simulink model "AC_DC"  (R2022b)
settings: Solver=FixedStepDiscrete  StartTime=0.0  StopTime=2  FixedStep=1e-6  RelTol=1e-3
libraries: spsRMSLib x11, spsSeriesRLCBranchLib x9, simulink x7, spsVoltageMeasurementLib x7, spsCurrentMeasurementLib x6, spsMosfetLib x6, spsIdealSwitchLib x3, spsFourierLib x2, spsMeanLib x2, slpidlib x2, sps_lib x1, spsControlledVoltageSourceLib x1
(part 1 of 2)
settings Model: SimulationMode=accelerator  Creator=XIAO  LastModifiedBy=XIAO
settings SolverCC: AutoInsertRateTranBlk=on
settings DataIOCC: ReturnWorkspaceOutputs=off

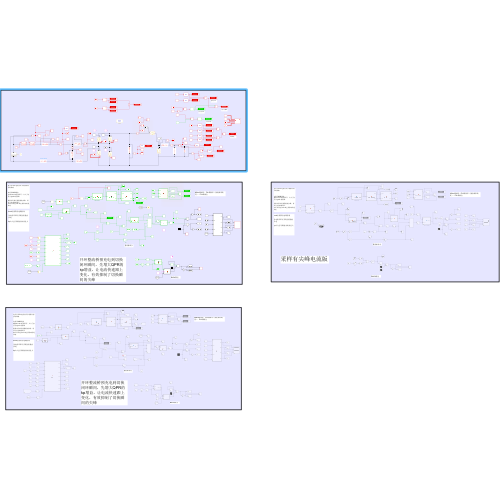
[thumbnail: Simulink's stored preview of the top-level diagram]
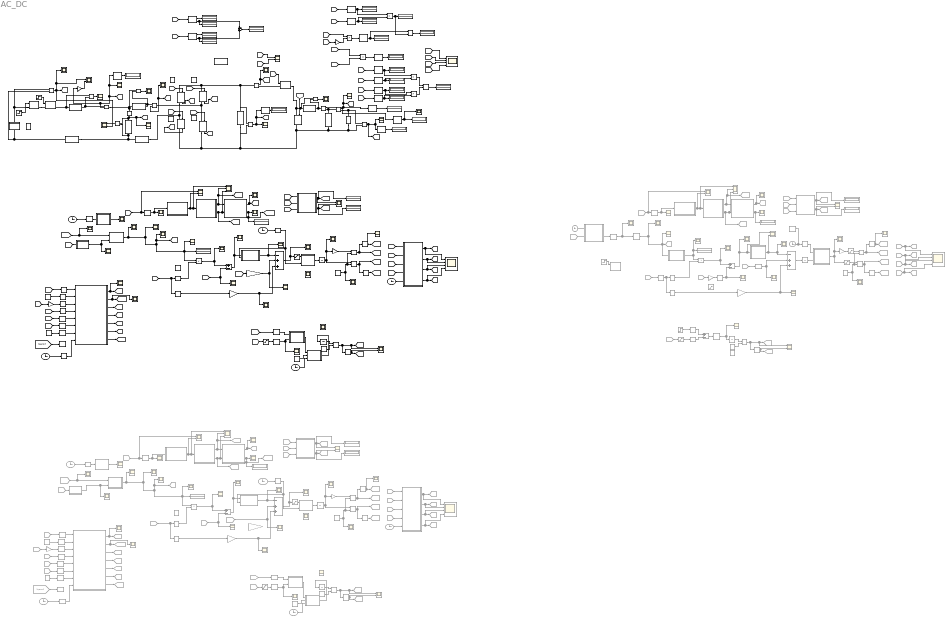
== system AC_DC ==
  note: BUCK降压
  note: buck恒流降压电路控制
      |
      | 单电流环即可实现恒流输出供电
      |
      | kp太大会导致输出纹波过大
  note: 功率因数PF
  note: 有功功率P
  note: 无功功率Q
  note: 视在功率s
  note: 电压外环PI 电流内环多谐振比例控制策略
      |
      | 电流环QPR调参
      | kp在0.2~0.3范围即可，太大了容易引起LCL谐振峰
      |
      | 根据实际情况调整谐波参数，谐波大对应kr就调大
      | wc可以固定在6~10主要影响的是带宽
  note: 效率η
  note: 整流桥部分
  note: 20khz锁相环，FLL锁频率（预防频率畸变），PLL锁相位
  note: 采样有尖峰电流版本
  note: 电压外环PI 电流内环多谐振比例控制策略
      |
      | 电流环QPR调参
      | kp在0.2~0.3范围即可，太大了容易引起LCL谐振峰
      |
      | 根据实际情况调整谐波参数，谐波大对应kr就调大
      | wc可以固定在6~10主要影响的是带宽
  note: buck恒流降压电路控制
      |
      | 单电流环即可实现恒流输出供电
      |
      | kp太大会导致输出纹波过大
  note: BUCK降压
  note: 整流桥部分
  note: 20khz锁相环，FLL锁频率（预防频率畸变），PLL锁相位
  note: 开环整流桥预充电到切换闭环瞬间，先增大QPR的kp增益，让电流快速跟上变化，有效抑制了切换瞬间的尖峰
  note: 电压外环PI 电流内环多谐振比例控制策略
      |
      | 电流环QPR调参
      | kp在0.2~0.3范围即可，太大了容易引起LCL谐振峰
      |
      | 根据实际情况调整谐波参数，谐波大对应kr就调大
      | wc可以固定在6~10主要影响的是带宽
  note: buck恒流降压电路控制
      |
      | 单电流环即可实现恒流输出供电
      |
      | kp太大会导致输出纹波过大
  note: BUCK降压
  note: 20khz锁相环，FLL锁频率（预防频率畸变），PLL锁相位
  note: 整流桥部分
  note: 开环整流桥预充电到切换闭环瞬间，先增大QPR的kp增益，让电流快速跟上变化，有效抑制了切换瞬间的尖峰
  -ug4 : Saturate  Commented=on  UpperLimit=1  LowerLimit=-1
  Add1 : Sum  Commented=on  Inputs=+-
  Add10 : Sum  Commented=on  Inputs=+-
  Add12 : Sum  Commented=on  Inputs=-++
  Add2 : Sum  Commented=on  Inputs=+-
  Add3 : Sum  Commented=on  Inputs=-++
  Add4 : Sum  Inputs=+-
  Add9 : Sum  Inputs=-++
  Clock{1..5} (5 alike) : Clock
  Clock{6..12} (7 alike) : Clock  Commented=on
  Constant{,4..6,8} (5 alike) : Constant  Value=0
  Constant1 : Constant  Commented=on  Value=0
  Constant10 : Constant  Commented=on  Value=55
  Constant11 : Constant  Commented=on
  Constant2 : Constant  Value=4.365
  Constant3 : Constant  Value=55
  Constant7 : Constant  Value=2
  Constant9 : Constant  Commented=on  Value=4.365
  Cos1 : Trigonometry  Operator=cos
  Cos2 : Trigonometry
  Cos3 : Trigonometry  Commented=on  Operator=cos
  Cos4 : Trigonometry  Commented=on
  Cos6 : Trigonometry  Commented=on  Operator=cos
  Cos7 : Trigonometry  Commented=on
  Current Measurement{1..6} (6 alike) : spsCurrentMeasurementLib/Current Measurement  PhasorSimulation=off  OutputType=Complex  PSBequivalent=0
  Display{,1..4,6..18,22,26..31} (25 alike) : Display
  Display{5,19..21,23,32..34} (8 alike) : Display  Commented=on
  Divide : Product  Inputs=*/
  Divide1 : Product  Inputs=/*
  Fourier7 : spsFourierLib/Fourier  Freq=50  n=1  InInit=[0, 0]  Ts=1e-6
  Fourier8 : spsFourierLib/Fourier  Freq=50  n=1  InInit=[0, 0]  Ts=1e-6
  From{19,41..42,55} (4 alike) : From  Commented=on  GotoTag=theta
  From43 : From  Commented=on  GotoTag=ua
  From{44,58,64,71} (4 alike) : From  Commented=on  GotoTag=Uref
  From45 : From  Commented=on  GotoTag=u_alpha
  From46 : From  Commented=on  GotoTag=u_beta
  From47 : From  Commented=on  GotoTag=IL2_
  From48 : From  Commented=on  GotoTag=ua_not
  From49 : From  Commented=on  GotoTag=ub_not
  From50 : From  Commented=on  GotoTag=IO_
  From51 : From  Commented=on  GotoTag=ub
  From52 : From  Commented=on  GotoTag=Uref_
  From53 : From  Commented=on  GotoTag=Udc_
  From54 : From  Commented=on  GotoTag=qerror
  From56 : From  Commented=on  GotoTag=Udc
  From57 : From  Commented=on  GotoTag=IL2
  From59 : From  Commented=on  GotoTag=ua
  From65 : From  Commented=on  GotoTag=u_alpha
  From66 : From  Commented=on  GotoTag=u_beta
  From67 : From  Commented=on  GotoTag=IL2
  From68 : From  Commented=on  GotoTag=ua_not
  From69 : From  Commented=on  GotoTag=ub_not
  From7 : From  Commented=on  GotoTag=IO
  From70 : From  Commented=on  GotoTag=ub
  From72 : From  Commented=on  GotoTag=Udc
  From73 : From  Commented=on  GotoTag=udc_target
  From74 : From  Commented=on  GotoTag=theat_
  From75 : From  Commented=on  GotoTag=IO
  From76 : From  Commented=on  GotoTag=I_target
  Gain{,1,8..9} (4 alike) : Gain  Gain=-1
  Gain2 : Gain  Gain=1/45.2544
  Gain{3..5,7} (4 alike) : Gain  Commented=on  Gain=-1
  Gain6 : Gain  Commented=on  Gain=1/45.2544
  Goto14 : Goto  Commented=on  GotoTag=theta
  Goto32 : Goto  Commented=on  GotoTag=u_q
  Goto38 : Goto  Commented=on  GotoTag=u_d
  Goto39 : Goto  Commented=on  GotoTag=u_alpha
  Goto40 : Goto  Commented=on  GotoTag=u_beta
  Goto41 : Goto  Commented=on  GotoTag=VT1
  Goto42 : Goto  Commented=on  GotoTag=VT2
  Goto43 : Goto  Commented=on  GotoTag=VT3
  Goto44 : Goto  Commented=on  GotoTag=VT4
  Goto45 : Goto  Commented=on  GotoTag=ub_not
  Goto46 : Goto  Commented=on  GotoTag=ub
  Goto47 : Goto  Commented=on  GotoTag=ua
  Goto48 : Goto  Commented=on  GotoTag=u_d
  Goto49 : Goto  Commented=on  GotoTag=u_alpha
  Goto50 : Goto  Commented=on  GotoTag=u_beta
  Goto51 : Goto  Commented=on  GotoTag=VT1
  Goto52 : Goto  Commented=on  GotoTag=VT2
  Goto53 : Goto  Commented=on  GotoTag=VT3
  Goto54 : Goto  Commented=on  GotoTag=VT4
  Goto55 : Goto  Commented=on  GotoTag=ua_not
  Goto56 : Goto  Commented=on  GotoTag=Igm
  Goto57 : Goto  Commented=on  GotoTag=ub_not
  Goto58 : Goto  Commented=on  GotoTag=ub
  Goto59 : Goto  Commented=on  GotoTag=ua
  Goto60 : Goto  Commented=on  GotoTag=ua_not
  Goto61 : Goto  Commented=on  GotoTag=PWM1
  Goto62 : Goto  Commented=on  GotoTag=PWM2
  Goto63 : Goto  Commented=on  GotoTag=Igm
  Goto64 : Goto  Commented=on  GotoTag=qerror
  Goto65 : Goto  Commented=on  GotoTag=Udc_
  Goto66 : Goto  Commented=on  GotoTag=udc_target
  Goto67 : Goto  Commented=on  GotoTag=IL2_
  Goto68 : Goto  Commented=on  GotoTag=Uref_
  Goto69 : Goto  Commented=on  GotoTag=theat_
  Goto70 : Goto  Commented=on  GotoTag=theta
  Goto71 : Goto  Commented=on  GotoTag=u_q
  Goto72 : Goto  Commented=on  GotoTag=IO_
  Goto73 : Goto  Commented=on  GotoTag=I_target
  Goto8 : Goto  Commented=on  GotoTag=PWM1
  Goto9 : Goto  Commented=on  GotoTag=PWM2
  Ideal Switch1 : spsIdealSwitchLib/Ideal Switch  Ron=0.001  Lon=0  IC=0  Rs=1e5  Cs=inf  Measurements=on
  Ideal Switch2 : spsIdealSwitchLib/Ideal Switch  Commented=on  Ron=0.001  Lon=0  IC=0  Rs=1e5  Cs=inf  Measurements=on
  Ideal Switch3 : spsIdealSwitchLib/Ideal Switch  Ron=0.001  Lon=0  IC=0  Rs=1e5  Cs=inf  Measurements=on
  MATLAB Function : MATLAB Function  TreatAsAtomicUnit=on
  MATLAB Function10 : MATLAB Function  Commented=on  TreatAsAtomicUnit=on
  MATLAB Function11 : MATLAB Function  TreatAsAtomicUnit=on
  MATLAB Function12 : MATLAB Function  TreatAsAtomicUnit=on
  MATLAB Function13 : MATLAB Function  Commented=on  TreatAsAtomicUnit=on
  MATLAB Function14 : MATLAB Function  Commented=on  TreatAsAtomicUnit=on
  MATLAB Function15 : MATLAB Function  Commented=on  TreatAsAtomicUnit=on
  MATLAB Function16 : MATLAB Function  TreatAsAtomicUnit=on
  MATLAB Function17 : MATLAB Function  Commented=on  TreatAsAtomicUnit=on
  MATLAB Function18 : MATLAB Function  Commented=on  TreatAsAtomicUnit=on
  MATLAB Function19 : MATLAB Function  Commented=on  TreatAsAtomicUnit=on
  MATLAB Function2 : MATLAB Function  Commented=on  TreatAsAtomicUnit=on
  MATLAB Function20 : MATLAB Function  Commented=on  TreatAsAtomicUnit=on
  MATLAB Function21 : MATLAB Function  Commented=on  TreatAsAtomicUnit=on
  MATLAB Function22 : MATLAB Function  Commented=on  TreatAsAtomicUnit=on
  MATLAB Function23 : MATLAB Function  Commented=on  TreatAsAtomicUnit=on
  MATLAB Function24 : MATLAB Function  Commented=on  TreatAsAtomicUnit=on
  MATLAB Function25 : MATLAB Function  Commented=on  TreatAsAtomicUnit=on
  MATLAB Function26 : MATLAB Function  Commented=on  TreatAsAtomicUnit=on
  MATLAB Function27 : MATLAB Function  Commented=on  TreatAsAtomicUnit=on
  MATLAB Function28 : MATLAB Function  Commented=on  TreatAsAtomicUnit=on
  MATLAB Function29 : MATLAB Function  TreatAsAtomicUnit=on
  MATLAB Function3 : MATLAB Function  TreatAsAtomicUnit=on
  MATLAB Function4 : MATLAB Function  TreatAsAtomicUnit=on
  MATLAB Function5 : MATLAB Function  TreatAsAtomicUnit=on
  MATLAB Function6 : MATLAB Function  TreatAsAtomicUnit=on
  MATLAB Function7 : MATLAB Function  TreatAsAtomicUnit=on
  MATLAB Function8 : MATLAB Function  TreatAsAtomicUnit=on
  MATLAB Function9 : MATLAB Function  TreatAsAtomicUnit=on
  Mean1 : spsMeanLib/Mean  Freq=50  Vinit=0  Ts=5e-5
  Mean2 : spsMeanLib/Mean  Freq=50  Vinit=0  Ts=5e-5
  Mosfet{,1..5} (6 alike) : spsMosfetLib/Mosfet  Ron=0.1  Lon=0  Rd=0.01  Vfd=0  IC=0  Rs=1e5  Cs=inf  Measurements=on
  NOT{1,5..9} (6 alike) : Logic  Commented=on  Operator=NOT  IconShape=distinctive  AllPortsSameDT=off  OutDataTypeStr=boolean
  NOT2 : Logic  Operator=NOT  IconShape=distinctive  AllPortsSameDT=off  OutDataTypeStr=boolean
  NOT3 : Logic  Operator=NOT  IconShape=distinctive  AllPortsSameDT=off  OutDataTypeStr=boolean
  NOT4 : Logic  Operator=NOT  IconShape=distinctive  AllPortsSameDT=off  OutDataTypeStr=boolean
  PID Controller1 : slpidlib/PID Controller  Commented=on  Controller=PI  Form=Parallel  TimeDomain=Discrete-time  UseExternalTs=off  SampleTime=-1  IntegratorMethod=Forward Euler  FilterMethod=Forward Euler  ControllerParametersSource=internal  P=1  I=10  UseKiTs=off  D=0  N=100  UseFilter=on  TunerSelectOption=Transfer Function Based (PID Tuner App)  InitialConditionSource=internal  InitialConditionForIntegrator=0  InitialConditionForFilter=0  DifferentiatorICPrevScaledInput=0  ExternalReset=none  TrackingMode=off  Kt=1  LimitOutput=off  SatLimitsSource=internal  UpperSaturationLimit=inf  LowerSaturationLimit=-inf  LinearizeAsGain=on  AntiWindupMode=none  Kb=1  LimitIntegrator=off  UpperIntegratorSaturationLimit=inf  LowerIntegratorSaturationLimit=-inf  POutMin=[]  POutMax=[]  IOutMin=[]  IOutMax=[]  DOutMin=[]  DOutMax=[]  NOutMin=[]  NOutMax=[]  SumOutMin=[]  SumOutMax=[]  SaturationOutMin=[]  SaturationOutMax=[]  PParamMin=[]  PParamMax=[]  IParamMin=[]  IParamMax=[]  DParamMin=[]  DParamMax=[]  NParamMin=[]  NParamMax=[]  KbParamMin=[]  KbParamMax=[]  KtParamMin=[]  KtParamMax=[]  KbOutMin=[]  KbOutMax=[]  KtOutMin=[]  KtOutMax=[]  IntegratorOutMin=[]  IntegratorOutMax=[]  FilterOutMin=[]  FilterOutMax=[]  SumI1OutMin=[]  SumI1OutMax=[]  SumI2OutMin=[]  SumI2OutMax=[]  SumI3OutMin=[]  SumI3OutMax=[]  SumI4OutMin=[]  SumI4OutMax=[]  SumDOutMin=[]  SumDOutMax=[]  DifferentiatorOutMin=[]  DifferentiatorOutMax=[]  FilterDiffOutCoefMin=[]  FilterDiffOutCoefMax=[]  ReciprocalOutMin=[]  ReciprocalOutMax=[]  SumDenOutMin=[]  SumDenOutMax=[]  SumNumOutMin=[]  SumNumOutMax=[]  DivideOutMin=[]  DivideOutMax=[]  UdiffTsProdOutMin=[]  UdiffTsProdOutMax=[]  NTsProdOutMin=[]  NTsProdOutMax=[]  UintegralTsProdOutMin=[]  UintegralTsProdOutMax=[]  UngainTsProdOutMin=[]  UngainTsProdOutMax=[]  ClampingZeroOutDataTypeStr=Inherit: Inherit via back propagation  ClampingZeroOutMin=[]  ClampingZeroOutMax=[]  FilterDenConstantOutDataTypeStr=Inherit: Inherit via back propagation  FilterDenConstantOutMin=[]  FilterDenConstantOutMax=[]  PCopyOutDataTypeStr=Inherit: Inherit via back propagation  PCopyOutMin=[]  PCopyOutMax=[]  NCopyOutDataTypeStr=Inherit: Inherit via back propagation  NCopyOutMin=[]  NCopyOutMax=[]  IntegratorContinuousStateAttributes=''  IntegratorStateMustResolveToSignalObject=off  IntegratorRTWStateStorageClass=Auto  FilterContinuousStateAttributes=''  FilterStateMustResolveToSignalObject=off  FilterRTWStateStorageClass=Auto  ParallelPVariant=InternalParameters  IdealPVariant=Disabled  IVariant=InternalParameters  DVariant=Disabled  IntegratorVariant=Discrete  SatVariant=Disabled  AWVariant=Passthrough  PCopyVariant=Disabled  TRVariant=Disabled  FdbkBlocksVariant=Forward  IdealPFdbkVariant=Disabled  SatFdbkVariant=Disabled  DerivativeFilterVariant=Disabled  NVariant=Disabled  NCopyVariant=Disabled_SignalSpec  FilterICVariant=Disabled  IntegratorICVariant=InternalICs  ExternalResetVariant=Disabled  TRSumVariant=Passthrough  SumFdbkVariant=Disabled  SumVariant=Sum_PI  TsampFilterVariant=InternalTs  TsampNgainVariant=Passthrough  TsampIntegralVariant=Passthrough  ExternalSaturationOutDataTypeStr=Inherit: Same as second input
  PID Controller3 : slpidlib/PID Controller  Commented=on  Controller=PI  Form=Parallel  TimeDomain=Discrete-time  UseExternalTs=off  SampleTime=-1  IntegratorMethod=Forward Euler  FilterMethod=Forward Euler  ControllerParametersSource=internal  P=0.5  I=10  UseKiTs=off  D=0  N=100  UseFilter=on  TunerSelectOption=Transfer Function Based (PID Tuner App)  InitialConditionSource=internal  InitialConditionForIntegrator=0  InitialConditionForFilter=0  DifferentiatorICPrevScaledInput=0  ExternalReset=none  TrackingMode=off  Kt=1  LimitOutput=off  SatLimitsSource=internal  UpperSaturationLimit=inf  LowerSaturationLimit=-inf  LinearizeAsGain=on  AntiWindupMode=none  Kb=1  LimitIntegrator=off  UpperIntegratorSaturationLimit=inf  LowerIntegratorSaturationLimit=-inf  POutMin=[]  POutMax=[]  IOutMin=[]  IOutMax=[]  DOutMin=[]  DOutMax=[]  NOutMin=[]  NOutMax=[]  SumOutMin=[]  SumOutMax=[]  SaturationOutMin=[]  SaturationOutMax=[]  PParamMin=[]  PParamMax=[]  IParamMin=[]  IParamMax=[]  DParamMin=[]  DParamMax=[]  NParamMin=[]  NParamMax=[]  KbParamMin=[]  KbParamMax=[]  KtParamMin=[]  KtParamMax=[]  KbOutMin=[]  KbOutMax=[]  KtOutMin=[]  KtOutMax=[]  IntegratorOutMin=[]  IntegratorOutMax=[]  FilterOutMin=[]  FilterOutMax=[]  SumI1OutMin=[]  SumI1OutMax=[]  SumI2OutMin=[]  SumI2OutMax=[]  SumI3OutMin=[]  SumI3OutMax=[]  SumI4OutMin=[]  SumI4OutMax=[]  SumDOutMin=[]  SumDOutMax=[]  DifferentiatorOutMin=[]  DifferentiatorOutMax=[]  FilterDiffOutCoefMin=[]  FilterDiffOutCoefMax=[]  ReciprocalOutMin=[]  ReciprocalOutMax=[]  SumDenOutMin=[]  SumDenOutMax=[]  SumNumOutMin=[]  SumNumOutMax=[]  DivideOutMin=[]  DivideOutMax=[]  UdiffTsProdOutMin=[]  UdiffTsProdOutMax=[]  NTsProdOutMin=[]  NTsProdOutMax=[]  UintegralTsProdOutMin=[]  UintegralTsProdOutMax=[]  UngainTsProdOutMin=[]  UngainTsProdOutMax=[]  ClampingZeroOutDataTypeStr=Inherit: Inherit via back propagation  ClampingZeroOutMin=[]  ClampingZeroOutMax=[]  FilterDenConstantOutDataTypeStr=Inherit: Inherit via back propagation  FilterDenConstantOutMin=[]  FilterDenConstantOutMax=[]  PCopyOutDataTypeStr=Inherit: Inherit via back propagation  PCopyOutMin=[]  PCopyOutMax=[]  NCopyOutDataTypeStr=Inherit: Inherit via back propagation  NCopyOutMin=[]  NCopyOutMax=[]  IntegratorContinuousStateAttributes=''  IntegratorStateMustResolveToSignalObject=off  IntegratorRTWStateStorageClass=Auto  FilterContinuousStateAttributes=''  FilterStateMustResolveToSignalObject=off  FilterRTWStateStorageClass=Auto  ParallelPVariant=InternalParameters  IdealPVariant=Disabled  IVariant=InternalParameters  DVariant=Disabled  IntegratorVariant=Discrete  SatVariant=Disabled  AWVariant=Passthrough  PCopyVariant=Disabled  TRVariant=Disabled  FdbkBlocksVariant=Forward  IdealPFdbkVariant=Disabled  SatFdbkVariant=Disabled  DerivativeFilterVariant=Disabled  NVariant=Disabled  NCopyVariant=Disabled_SignalSpec  FilterICVariant=Disabled  IntegratorICVariant=InternalICs  ExternalResetVariant=Disabled  TRSumVariant=Passthrough  SumFdbkVariant=Disabled  SumVariant=Sum_PI  TsampFilterVariant=InternalTs  TsampNgainVariant=Passthrough  TsampIntegralVariant=Passthrough  ExternalSaturationOutDataTypeStr=Inherit: Same as second input
  Product{,1..5} (6 alike) : Product
  Product11 : Product  Commented=on
  Product6 : Product  Commented=on
  RMS{,3..8} (7 alike) : spsRMSLib/RMS  TrueRMS=on  Freq=50  RMSInit=24  Ts=1e-6
  RMS{1..2,9..10} (4 alike) : spsRMSLib/RMS  TrueRMS=on  Freq=50  RMSInit=120  Ts=1e-6
  Relational Operator1 : RelationalOperator  Commented=on  OutDataTypeStr=boolean  RndMeth=Simplest  InputSameDT=off
  Relational Operator2 : RelationalOperator  OutDataTypeStr=boolean  RndMeth=Simplest  InputSameDT=off
  Relational Operator3 : RelationalOperator  Commented=on  OutDataTypeStr=boolean  RndMeth=Simplest  InputSameDT=off
  Repeating Sequence1 : simulink/Sources/Repeating Sequence  Commented=on  rep_seq_t=[0 0.0001]  rep_seq_y=[0 1 ]
  Repeating Sequence2 : simulink/Sources/Repeating Sequence  Commented=on  rep_seq_t=[0 0.00005 0.0001]  rep_seq_y=[0 1 0]
  Repeating Sequence3 : simulink/Sources/Repeating Sequence  Commented=on  rep_seq_t=[0 0.00005 0.0001]  rep_seq_y=[0 1 0]
  Repeating Sequence4 : simulink/Sources/Repeating Sequence  Commented=on  rep_seq_t=[0, 5e-5, 1e-4]  rep_seq_y=[-1, 1, -1]
  Repeating Sequence5 : simulink/Sources/Repeating Sequence  rep_seq_t=[0 0.00005 0.0001]  rep_seq_y=[0 1 0]
  Repeating Sequence6 : simulink/Sources/Repeating Sequence  rep_seq_t=[0, 5e-5, 1e-4]  rep_seq_y=[-1, 1, -1]
  Repeating Sequence7 : simulink/Sources/Repeating Sequence  Commented=on  rep_seq_t=[0, 5e-5, 1e-4]  rep_seq_y=[-1, 1, -1]
  Scope : Scope  NumInputPorts=4
  Scope{1..3,5..7,11..15,18..20,22,24..31,38..42,44..47,81,85..86} (35 alike) : Scope
  Scope{4,10,32..34,43,48..52,54,57..60,62..68,70,72..79,82..83,87..92} (40 alike) : Scope  Commented=on
  Scope{8,16,21,37,93} (5 alike) : Scope  NumInputPorts=2
  Scope17 : Scope  NumInputPorts=3
  Scope23 : Scope  NumInputPorts=4
  Scope{9,35,53,56,69,80,84} (7 alike) : Scope  Commented=on  NumInputPorts=2
  Scope36 : Scope  Commented=on  NumInputPorts=3
  Scope55 : Scope  Commented=on  NumInputPorts=4
  Scope61 : Scope  Commented=on  NumInputPorts=3
  Scope71 : Scope  Commented=on  NumInputPorts=4
  Series RLC Branch : spsSeriesRLCBranchLib/Series RLC Branch  LConnTagsString=__new0  RConnTagsString=__new0  BranchType=RL  Resistance=0.1  Inductance=2.5e-3  SetiL0=off  InitialCurrent=0  Capacitance=1e-6  Setx0=off  InitialVoltage=0  Measurements=None
  Series RLC Branch1 : spsSeriesRLCBranchLib/Series RLC Branch  LConnTagsString=__new0  RConnTagsString=__new0  BranchType=C  Resistance=0  Inductance=1e-3  SetiL0=off  InitialCurrent=0  Capacitance=940e-6  Setx0=off  InitialVoltage=0  Measurements=None
  Series RLC Branch2 : spsSeriesRLCBranchLib/Series RLC Branch  LConnTagsString=__new0  RConnTagsString=__new0  BranchType=R  Resistance=12  Inductance=1e-3  SetiL0=off  InitialCurrent=0  Capacitance=1000e-6  Setx0=off  InitialVoltage=0  Measurements=None
  Series RLC Branch3 : spsSeriesRLCBranchLib/Series RLC Branch  LConnTagsString=__new0  RConnTagsString=__new0  BranchType=RL  Resistance=0.1  Inductance=0.00012  SetiL0=off  InitialCurrent=0  Capacitance=220e-6  Setx0=off  InitialVoltage=0  Measurements=None
  Series RLC Branch4 : spsSeriesRLCBranchLib/Series RLC Branch  LConnTagsString=__new0  RConnTagsString=__new0  BranchType=RL  Resistance=0.1  Inductance=0.0015  SetiL0=off  InitialCurrent=0  Capacitance=220e-6  Setx0=off  InitialVoltage=0  Measurements=None
  Series RLC Branch5 : spsSeriesRLCBranchLib/Series RLC Branch  LConnTagsString=__new0  RConnTagsString=__new0  BranchType=RL  Resistance=0.1  Inductance=0.0015  SetiL0=off  InitialCurrent=0  Capacitance=220e-6  Setx0=off  InitialVoltage=0  Measurements=None
  Series RLC Branch6 : spsSeriesRLCBranchLib/Series RLC Branch  LConnTagsString=__new0  RConnTagsString=__new0  BranchType=RL  Resistance=0.1  Inductance=0.00012  SetiL0=off  InitialCurrent=0  Capacitance=220e-6  Setx0=off  InitialVoltage=0  Measurements=None
  Series RLC Branch7 : spsSeriesRLCBranchLib/Series RLC Branch  LConnTagsString=__new0  RConnTagsString=__new0  BranchType=RC  Resistance=0.1  Inductance=0  SetiL0=off  InitialCurrent=0  Capacitance=10e-6  Setx0=off  InitialVoltage=0  Measurements=None
  Series RLC Branch9 : spsSeriesRLCBranchLib/Series RLC Branch  LConnTagsString=__new0  RConnTagsString=__new0  BranchType=RC  Resistance=0.01  Inductance=0  SetiL0=off  InitialCurrent=0  Capacitance=1880e-6  Setx0=off  InitialVoltage=0  Measurements=None
  Step1 : Step  Commented=on  Time=0.15  After=2  SampleTime=1e-6
  Step2 : Step  Commented=on  Time=0.15  SampleTime=1e-6
  Step3 : Step  Time=1.75  Before=1  After=0  SampleTime=1e-6
  Step4 : Step  Time=0  SampleTime=1e-6
  Sum4 : Sum  Inputs=+-
  Unit Delay{1,3,5..6} (4 alike) : UnitDelay  Commented=on  SampleTime=5e-5  HasFrameUpgradeWarning=on
  Unit Delay2 : UnitDelay  SampleTime=5e-5  HasFrameUpgradeWarning=on
  Unit Delay4 : UnitDelay  SampleTime=5e-5  HasFrameUpgradeWarning=on
  Voltage Measurement{,1..6} (7 alike) : spsVoltageMeasurementLib/Voltage Measurement  PhasorSimulation=off  OutputType=Complex  PSBequivalent=0
  WL1 : Gain  Gain=0.471
  WL2 : Gain  Commented=on  Gain=0.471
  WL3 : Gain  Commented=on  Gain=0.471
  Zero-Order Hold{1,8,13,17..33,36..38} (23 alike) : ZeroOrderHold  Commented=on  SampleTime=5e-5
  Zero-Order Hold{2..7,9..12,14..16,39} (14 alike) : ZeroOrderHold  SampleTime=5e-5
  i1 : Scope  NumInputPorts=2
  i3 : Scope
  iL1 : Scope  NumInputPorts=2
  iL10 : Scope  Commented=on  NumInputPorts=2
  iL2 : Scope  Commented=on  NumInputPorts=2
  powergui : sps_lib/powergui  Priority=1  SimulationMode=Discrete  SampleTime=1e-6  frequency=60  Iterations=50  frequencyindice=0  Pbase=100e6  ErrMax=1e-4  UnitsV=kV  UnitsW=MW  buscounter=0  FunctionMessages=off  echomessages=off  EnableUseOfTLC=off  CurrentSourceSwitches=off  DisableSnubberDevices=off  DisableRonSwitches=off  DisableVfSwitches=off  DisplayEquations=off  AutomaticDiscreteSolvers=off  SolverType=Tustin/Backward Euler (TBE)  Interpol=off  ExternalGateDelay=off  methode=off  Ts=100  x0status=blocks  SPID=on  SwTol=0  HookPort=off  NonlinearTolerance=1e-4  nMaxIteration=100  ContinueOnMaxIteration=off  RestoreLinks=warning  ResistiveCurrentMeasurement=off  Frange=[0:2:500]  Ylog=off  Xlog=on  ShowGrid=off  save=off  variable=ZData  structure=0  ZoomFFT=off  StartTime=0.0  cycles=1  DisplayStyle=1  fundamental=60  FreqAxis=off  MaxFrequency=1000  frequencyindicesteady=1  RmsSteady=1  display=off
  ua1 : RelationalOperator  Operator=>  OutDataTypeStr=boolean  RndMeth=Simplest  InputSameDT=off
  ua2 : RelationalOperator  Commented=on  Operator=>  OutDataTypeStr=boolean  RndMeth=Simplest  InputSameDT=off
  ua4 : RelationalOperator  Commented=on  Operator=>  OutDataTypeStr=boolean  RndMeth=Simplest  InputSameDT=off
  ub1 : RelationalOperator  Operator=>  OutDataTypeStr=boolean  RndMeth=Simplest  InputSameDT=off
  ub2 : RelationalOperator  Commented=on  Operator=>  OutDataTypeStr=boolean  RndMeth=Simplest  InputSameDT=off
  ub4 : RelationalOperator  Commented=on  Operator=>  OutDataTypeStr=boolean  RndMeth=Simplest  InputSameDT=off
  ug1 : Saturate  Commented=on  UpperLimit=0.98  LowerLimit=-0.98
  ug2 : Saturate  UpperLimit=0.98  LowerLimit=-0.98
  ug3 : Saturate  Commented=on  UpperLimit=5  LowerLimit=-5
  ug4 : Saturate  Commented=on  UpperLimit=1  LowerLimit=-1
  ug5 : Saturate  Commented=on  UpperLimit=5  LowerLimit=-5
  ug6 : Saturate  Commented=on  UpperLimit=5  LowerLimit=-5
  ug7 : Saturate  UpperLimit=5  LowerLimit=-5
  合闸后再传入信号1 : MATLAB Function  Commented=on  TreatAsAtomicUnit=on
  带有谐波的电网 : Subsystem
  模仿开关控制3 : MATLAB Function  Commented=on  TreatAsAtomicUnit=on
  理想电网 : spsACVoltageSourceLib/AC Voltage Source  Amplitude=32*1.414  Phase=0  Frequency=50  SampleTime=0  Measurements=None  BusType=swing  Pref=10e3  Qref=0  Qmin=-inf  Qmax=+inf
  级联谐波抑制1 : MATLAB Function  TreatAsAtomicUnit=on
  级联谐波抑制2 : MATLAB Function  Commented=on  TreatAsAtomicUnit=on
  级联谐波抑制4 : MATLAB Function  Commented=on  TreatAsAtomicUnit=on
  wires:
  Voltage Measurement1/1 -> [U_O], RMS2/1, Scope5/1
  RMS2/1 -> Display2/1
  Current Measurement1/1 -> RMS1/1, Scope2/1, [IO]
  [PWM2] -> Mosfet1/1
  RMS1/1 -> Display1/1
  [PWM1] -> Mosfet/1
  [Uref] -> Fourier7/1
  [IL2] -> Scope8/2
  Voltage Measurement/1 -> [Udc], RMS4/1, Scope7/1
  RMS4/1 -> Display4/1
  [M2] -> Scope/2
  Current Measurement2/1 -> i3/1, [I_c]
  Fourier7/1 -> Display31/1
  RMS3/1 -> Product1/1, Display3/1
  Product/1 -> Mean1/1
  Mean1/1 -> Divide/1, Display12/1
  [M1] -> Scope/1
  Fourier8/1 -> Display28/1
  Fourier8/2 -> Sum4/2, Display29/1
  Sum4/1 -> Display30/1
  Mean2/1 -> Display26/1
  [IL2] -> Product2/1
  Zero-Order Hold29/1 -> Add10/2, Scope64/1
  Gain7/1 -> -ug4/1
  [M4] -> Scope/4
  Repeating Sequence4/1 -> ub4/2, ua4/2, Scope53/1
  PID Controller3/1 -> Scope59/1, MATLAB Function15/1(IGm_total), Goto63/1, Scope57/1
  Zero-Order Hold25/1 -> Cos7/1, Cos6/1
  Voltage Measurement3/1 -> i1/1
  [IL1] -> RMS/1
  Zero-Order Hold28/1 -> PID Controller3/1, Scope63/1
  合闸后再传入信号1/2(Udc_error) -> Zero-Order Hold28/1
  Mosfet5/1 -> [M2]
  [M3] -> Scope/3
  NOT8/1 -> Goto60/1
  MATLAB Function15/1(Igm_clean) -> Scope58/1, Display5/1, Product11/1
  Fourier7/2 -> Display27/1, Sum4/1
  Mosfet2/1 -> [M3]
  -ug4/1 -> ub4/1
  From71/1 -> Zero-Order Hold31/1
  [u_beta] -> Product2/2
  Current Measurement3/1 -> [IL1], RMS10/1, Scope3/1, Gain8/1
  Current Measurement5/1 -> Scope6/1, [Idc]
  模仿开关控制3/1(mod_out) -> ug4/1, Scope52/1, Gain7/1
  ua4/1 -> Goto59/1, NOT8/1
  ug4/1 -> ua4/1
  Divide/1 -> Display14/1
  Clock7/1 -> 合闸后再传入信号1/1(t)
  Unit Delay3/1 -> 模仿开关控制3/2(mod_in)
  [Uref] -> Product/1
  Cos6/1 -> Product11/2
  From55/1 -> Zero-Order Hold25/1
  Add12/1 -> Unit Delay3/1
  [Uref] -> Scope8/1
  Product2/1 -> Mean2/1
  Cos7/1 -> WL3/1
  [IL2] -> Fourier8/1
  From59/1 -> Scope55/1, Goto51/1
  Mosfet4/1 -> [M1]
  Voltage Measurement2/1 -> i1/2, Scope93/1, Scope81/1, [Uref]
  Product1/1 -> Divide/2, Display13/1
  From72/1 -> 合闸后再传入信号1/2(Udc)
  From70/1 -> Scope55/3, Goto53/1
  Mosfet3/1 -> [M4]
  From69/1 -> Scope55/4, Goto54/1
  [IL1] -> Gain9/1
  NOT7/1 -> Scope54/1, Goto57/1
  RMS/1 -> Product1/2, Display/1
  [Uref] -> RMS3/1
  ub4/1 -> Goto58/1, NOT7/1
  Zero-Order Hold31/1 -> Add12/2, Scope50/1
  MATLAB Function20/1(m) -> Scope84/2, Scope60/1, Add12/1
  WL3/1 -> Add12/3, Scope32/1
  Clock8/1 -> Zero-Order Hold37/1, Zero-Order Hold38/1
  Product11/1 -> Add10/1, Scope62/1
  From68/1 -> Scope55/2, Goto52/1
  Zero-Order Hold1/1 -> Add1/2
  NOT1/1 -> Goto9/1, Scope9/2
  PID Controller1/1 -> Unit Delay1/1, Scope10/1
  Relational Operator1/1 -> NOT1/1, Scope9/1, Goto8/1
  Add1/1 -> PID Controller1/1
  Repeating Sequence3/1 -> Relational Operator1/2
  Unit Delay1/1 -> Relational Operator1/1
  From7/1 -> ug5/1
  Step1/1 -> Zero-Order Hold36/1
  [Uref] -> RMS6/1
  RMS5/1 -> Display6/1, Product3/2
  RMS6/1 -> Product3/1, Display9/1
  [IL1] -> RMS5/1
  [U_O] -> RMS7/1
  [IO] -> RMS8/1
  RMS7/1 -> Product4/1, Display10/1
  RMS8/1 -> Product4/2, Display11/1
  Product3/1 -> Divide1/1
  Product4/1 -> Divide1/2
  Divide1/1 -> Display15/1
  MATLAB Function2/2(qerror) -> Scope4/1, Display32/1
  From66/1 -> MATLAB Function10/2(beta)
  From65/1 -> MATLAB Function10/1(alpha)
  MATLAB Function19/1(alpha) -> Scope36/2, Goto49/1, MATLAB Function2/1(u_alpha)
  MATLAB Function10/1(d) -> iL10/1, Display34/1, Goto48/1
  From64/1 -> Scope35/1, Zero-Order Hold20/1
  MATLAB Function2/1(theta) -> Scope33/1, Goto14/1
  From19/1 -> MATLAB Function10/3(theta)
  级联谐波抑制4/1(y) -> Scope35/2, Scope36/1, MATLAB Function19/1(uin)
  Zero-Order Hold20/1 -> 级联谐波抑制4/1(u), Scope34/1
  MATLAB Function10/2(q) -> Display33/1, Goto32/1, iL10/2
  MATLAB Function19/2(beta) -> Scope36/3, MATLAB Function2/2(u_beta), Goto50/1
  Step2/1 -> Ideal Switch2/1
  Add10/1 -> Scope65/1, Scope84/1, MATLAB Function20/1(i_error)
  ug5/1 -> Zero-Order Hold1/1
  Zero-Order Hold36/1 -> Add1/1
  Zero-Order Hold38/1 -> 模仿开关控制3/1(t)
  From67/1 -> Gain3/1
  Product5/1 -> Add4/1, Scope28/1
  [IL2_] -> Add4/2, Scope30/1
  Clock3/1 -> Zero-Order Hold14/1
  MATLAB Function5/1(alpha) -> [u_alpha], Scope17/2, MATLAB Function6/1(u_alpha)
  MATLAB Function6/2(qerror) -> [qerror], Display16/1, Scope18/1
  Zero-Order Hold14/1 -> MATLAB Function8/1(t)
  ug7/1 -> Zero-Order Hold9/1
  Unit Delay4/1 -> ua1/1, Scope20/1, Gain1/1
  MATLAB Function16/5(out5) -> [theat_]
  MATLAB Function5/2(beta) -> Scope17/3, MATLAB Function6/2(u_beta), [u_beta]
  Relational Operator2/1 -> NOT2/1, Scope37/1, [PWM1]
  MATLAB Function29/1(m) -> Add9/1, Scope27/1
  Gain1/1 -> ub1/1
  [udc_target] -> MATLAB Function12/1(I_ref), Scope41/1
  Add9/1 -> ug2/1, Scope38/1
  [Uref] -> Scope16/1, Zero-Order Hold10/1
  WL1/1 -> Add9/3, Scope13/1
  Zero-Order Hold11/1 -> MATLAB Function7/3(t)
  MATLAB Function16/1(out1) -> Scope39/1, [Udc_]
  MATLAB Function6/1(theta) -> Scope14/1, [theta]
  [IO_] -> ug7/1
  Repeating Sequence5/1 -> Relational Operator2/2
  Zero-Order Hold10/1 -> 级联谐波抑制1/1(u), Scope15/1
  [theta] -> MATLAB Function3/3(theta)
  MATLAB Function3/2(q) -> Display17/1, [u_q], iL1/2
  Zero-Order Hold12/1 -> MATLAB Function16/8(t)
  Zero-Order Hold4/1 -> MATLAB Function16/3(in3)
  级联谐波抑制1/1(y) -> Scope16/2, Scope17/1, MATLAB Function5/1(uin)
  [theta] -> Zero-Order Hold6/1
  [theat_] -> Cos2/1, Cos1/1
  Clock2/1 -> Zero-Order Hold11/1
  [Uref] -> Zero-Order Hold5/1
  MATLAB Function16/3(out3) -> [IL2_]
  [qerror] -> Zero-Order Hold7/1
  MATLAB Function16/4(out4) -> [Uref_]
  Zero-Order Hold6/1 -> MATLAB Function16/5(in5)
  MATLAB Function16/2(out2) -> Scope40/1, [udc_target]
  Zero-Order Hold3/1 -> MATLAB Function16/2(in2)
  [IL2] -> Gain/1
  MATLAB Function16/6(out6) -> [IO_]
  MATLAB Function16/7(out7) -> [I_target]
  NOT3/1 -> Scope22/1, [ub_not]
  Zero-Order Hold5/1 -> MATLAB Function16/4(in4)
  NOT4/1 -> [ua_not]
  Unit Delay2/1 -> Relational Operator2/1
  [u_alpha] -> MATLAB Function3/1(alpha)
  MATLAB Function3/1(d) -> iL1/1, Display7/1, [u_d]
  [IO] -> Zero-Order Hold39/1
  Constant3/1 -> Zero-Order Hold3/1
  Cos2/1 -> WL1/1
  NOT2/1 -> [PWM2], Scope37/2
  Cos1/1 -> Product5/2
  [u_beta] -> MATLAB Function3/2(beta)
  Zero-Order Hold9/1 -> MATLAB Function4/2(I_fb), Scope86/1
  [I_target] -> Zero-Order Hold15/1
  Constant7/1 -> Zero-Order Hold16/1
  ub1/1 -> [ub], NOT3/1
  Zero-Order Hold16/1 -> MATLAB Function16/7(in7)
  Repeating Sequence6/1 -> ub1/2, ua1/2, Scope21/1
  [Udc] -> Zero-Order Hold2/1
  MATLAB Function8/1(utarget) -> Scope42/1
  ua1/1 -> [ua], NOT4/1
  MATLAB Function12/1(duty_out) -> Product5/1, Scope25/1, Display8/1, [Igm], Scope26/1, Scope24/1, Scope29/1
  Clock1/1 -> Zero-Order Hold12/1
  [Uref_] -> Gain2/1
  Add4/1 -> MATLAB Function29/1(i_error), Scope31/1
  Zero-Order Hold39/1 -> MATLAB Function16/6(in6)
  Zero-Order Hold2/1 -> MATLAB Function16/1(in1)
  Step3/1 -> Ideal Switch1/1
  Current Measurement6/1 -> RMS9/1
  Voltage Measurement4/1 -> Scope44/1
  Voltage Measurement5/1 -> Scope45/1
  Voltage Measurement6/1 -> Scope46/1
  MATLAB Function7/1(y) -> Unit Delay4/1
  Constant/1 -> MATLAB Function9/2(in2)
  MATLAB Function9/1(y) -> Unit Delay2/1
  Clock4/1 -> MATLAB Function9/3(t)
  [ua] -> MATLAB Function/1(ua)
  [ua_not] -> MATLAB Function/2(uanot)
  [ub] -> MATLAB Function/3(ub)
  [ub_not] -> MATLAB Function/4(ubnot)
  Clock5/1 -> MATLAB Function/5(t)
  MATLAB Function/4(VT4) -> Scope23/4, [VT4]
  MATLAB Function/3(VT3) -> Scope23/3, [VT3]
  MATLAB Function/2(VT2) -> Scope23/2, [VT2]
  MATLAB Function/1(VT1) -> Scope23/1, [VT1]
  ug2/1 -> MATLAB Function7/1(in1)
  [Udc_] -> MATLAB Function11/1(IGm_total)
  RMS9/1 -> Scope1/1, Display22/1
  Current Measurement4/1 -> Scope12/1, [IL2]
  Gain3/1 -> Zero-Order Hold29/1
  [VT4] -> Mosfet3/1
  [VT3] -> Mosfet2/1
  [VT1] -> Mosfet4/1
  [VT2] -> Mosfet5/1
  Gain/1 -> Zero-Order Hold4/1
  MATLAB Function11/1(IGm_clean) -> MATLAB Function12/2(I_fb), Scope47/1
  Zero-Order Hold15/1 -> MATLAB Function4/1(I_ref)
  MATLAB Function4/1(duty_out) -> MATLAB Function9/1(in1)
  Step4/1 -> Ideal Switch3/1
  RMS10/1 -> Display18/1
  Zero-Order Hold19/1 -> MATLAB Function23/1(I_ref)
  MATLAB Function17/1(IGm_clean) -> Scope90/1, MATLAB Function18/2(I_fb)
  Gain4/1 -> Zero-Order Hold26/1
  MATLAB Function23/1(duty_out) -> MATLAB Function28/1(in1)
  From49/1 -> MATLAB Function13/4(ubnot)
  Zero-Order Hold24/1 -> MATLAB Function21/6(in6)
  MATLAB Function26/1(y) -> Unit Delay6/1
  Zero-Order Hold33/1 -> MATLAB Function23/2(I_fb), Scope92/1
  ug1/1 -> MATLAB Function26/1(in1)
  ug6/1 -> Zero-Order Hold33/1
  From41/1 -> MATLAB Function22/3(theta)
  MATLAB Function14/1(m) -> Add3/1, Scope75/1
  MATLAB Function21/2(out2) -> Scope87/1, Goto66/1
  Constant1/1 -> MATLAB Function28/2(in2)
  NOT9/1 -> Goto55/1
  From44/1 -> Scope56/1, Zero-Order Hold8/1
  From57/1 -> Gain4/1
  Repeating Sequence2/1 -> Relational Operator3/2
  MATLAB Function21/3(out3) -> Goto67/1
  From54/1 -> Zero-Order Hold32/1
  From58/1 -> Zero-Order Hold27/1
  MATLAB Function25/2(qerror) -> Goto64/1, Display19/1, Scope66/1
  MATLAB Function22/2(q) -> Display20/1, Goto71/1, iL2/2
  Relational Operator3/1 -> NOT5/1, Scope80/1, Goto61/1
  Zero-Order Hold8/1 -> 级联谐波抑制2/1(u), Scope51/1
  Zero-Order Hold13/1 -> MATLAB Function14/2(t), MATLAB Function26/3(t)
  MATLAB Function25/1(theta) -> Scope49/1, Goto70/1
  MATLAB Function21/1(out1) -> Scope83/1, Goto65/1
  From73/1 -> MATLAB Function18/1(I_ref), Scope88/1
  MATLAB Function21/5(out5) -> Goto69/1
  Add3/1 -> ug1/1, Scope82/1
  Constant10/1 -> Zero-Order Hold23/1
  From45/1 -> MATLAB Function22/1(alpha)
  From75/1 -> Zero-Order Hold24/1
  Unit Delay5/1 -> Relational Operator3/1
  NOT6/1 -> Scope70/1, Goto45/1
  Constant11/1 -> Zero-Order Hold21/1
  MATLAB Function13/2(VT2) -> Scope71/2, Goto42/1
  Zero-Order Hold18/1 -> MATLAB Function27/1(t)
  MATLAB Function22/1(d) -> iL2/1, Display21/1, Goto38/1
  Product6/1 -> Add2/1, Scope76/1
  Zero-Order Hold21/1 -> MATLAB Function21/7(in7)
  Zero-Order Hold30/1 -> MATLAB Function21/5(in5)
  From51/1 -> MATLAB Function13/3(ub)
  MATLAB Function21/7(out7) -> Goto73/1
  From48/1 -> MATLAB Function13/2(uanot)
  NOT5/1 -> Goto62/1, Scope80/2
  Clock10/1 -> Zero-Order Hold18/1
  Gain5/1 -> ub2/1
  From74/1 -> Cos4/1, Cos3/1
  Repeating Sequence7/1 -> ub2/2, ua2/2, Scope69/1
  From50/1 -> ug6/1
  WL2/1 -> Add3/3, Scope48/1
  Add2/1 -> MATLAB Function14/1(i_error), Scope79/1
  MATLAB Function13/1(VT1) -> Scope71/1, Goto41/1
  Clock12/1 -> MATLAB Function13/5(t)
  Unit Delay6/1 -> ua2/1, Scope68/1, Gain5/1
  From42/1 -> Zero-Order Hold30/1
  From43/1 -> MATLAB Function13/1(ua)
  MATLAB Function13/3(VT3) -> Scope71/3, Goto43/1
  Clock11/1 -> MATLAB Function28/3(t)
  MATLAB Function21/6(out6) -> Goto72/1
  Clock6/1 -> Zero-Order Hold17/1
  ub2/1 -> Goto46/1, NOT6/1
  Zero-Order Hold17/1 -> MATLAB Function21/8(t)
  From52/1 -> Add3/2, Scope67/1
  Zero-Order Hold27/1 -> MATLAB Function21/4(in4)
  MATLAB Function13/4(VT4) -> Scope71/4, Goto44/1
  From47/1 -> Add2/2, Scope78/1
  Zero-Order Hold22/1 -> MATLAB Function21/1(in1)
  MATLAB Function21/4(out4) -> Goto68/1
  MATLAB Function24/2(beta) -> Scope61/3, MATLAB Function25/2(u_beta), Goto40/1
  From53/1 -> MATLAB Function17/1(IGm_total)
  MATLAB Function28/1(y) -> Unit Delay5/1
  级联谐波抑制2/1(y) -> Scope56/2, Scope61/1, MATLAB Function24/1(uin)
  MATLAB Function27/1(utarget) -> Scope89/1
  Cos3/1 -> Product6/2
  From76/1 -> Zero-Order Hold19/1
  Zero-Order Hold23/1 -> MATLAB Function21/2(in2)
  MATLAB Function18/1(duty_out) -> Product6/1, Scope73/1, Display23/1, Goto56/1, Scope74/1, Scope72/1, Scope77/1
  From56/1 -> Zero-Order Hold22/1
  From46/1 -> MATLAB Function22/2(beta)
  Cos4/1 -> WL2/1
  Zero-Order Hold26/1 -> MATLAB Function21/3(in3)
  ua2/1 -> Goto47/1, NOT9/1
  MATLAB Function24/1(alpha) -> Goto39/1, Scope61/2, MATLAB Function25/1(u_alpha)
  Clock9/1 -> Zero-Order Hold13/1
  Gain2/1 -> Scope19/1, Add9/2
  Gain8/1 -> Scope93/2
  Gain9/1 -> Product/2
  connections:
  Series RLC Branch/LConn1 -- Mosfet/RConn1 -- Mosfet1/LConn1 -- Voltage Measurement6/LConn1
  Series RLC Branch1/LConn1 -- Current Measurement6/LConn1 -- Current Measurement1/RConn1
  Current Measurement2/LConn1 -- Series RLC Branch5/RConn1 -- Voltage Measurement5/LConn1 -- Current Measurement3/LConn1
  Series RLC Branch2/RConn1 -- Voltage Measurement1/LConn2 -- Series RLC Branch1/RConn1 -- Series RLC Branch9/RConn1 -- Voltage Measurement/LConn2 -- Mosfet5/RConn1 -- Mosfet3/RConn1 -- Mosfet1/RConn1
  Mosfet2/RConn1 -- Series RLC Branch4/LConn1 -- Mosfet3/LConn1
  Mosfet4/LConn1 -- Mosfet2/LConn1 -- Voltage Measurement/LConn1 -- Series RLC Branch9/LConn1 -- Current Measurement5/LConn1
  Current Measurement2/RConn1 -- Voltage Measurement3/LConn1 -- Series RLC Branch7/LConn1
  Series RLC Branch5/LConn1 -- Voltage Measurement5/LConn2 -- Current Measurement4/RConn1
  Mosfet/LConn1 -- Current Measurement5/RConn1
  Mosfet5/LConn1 -- Current Measurement4/LConn1 -- Mosfet4/RConn1
  Current Measurement1/LConn1 -- Voltage Measurement6/LConn2 -- Series RLC Branch/RConn1
  Series RLC Branch6/RConn1 -- Voltage Measurement4/LConn1 -- Ideal Switch1/RConn1
  Current Measurement6/RConn1 -- Voltage Measurement1/LConn1 -- Series RLC Branch2/LConn1
  Voltage Measurement4/LConn2 -- Current Measurement3/RConn1 -- Series RLC Branch6/LConn1
  Voltage Measurement2/LConn2 -- Series RLC Branch3/RConn1 -- 带有谐波的电网/LConn1
  Voltage Measurement3/LConn2 -- Series RLC Branch7/RConn1 -- Series RLC Branch3/LConn1 -- Series RLC Branch4/RConn1
  带有谐波的电网/RConn1 -- Ideal Switch3/LConn1 -- Voltage Measurement2/LConn1
  Ideal Switch3/RConn1 -- Ideal Switch1/LConn1

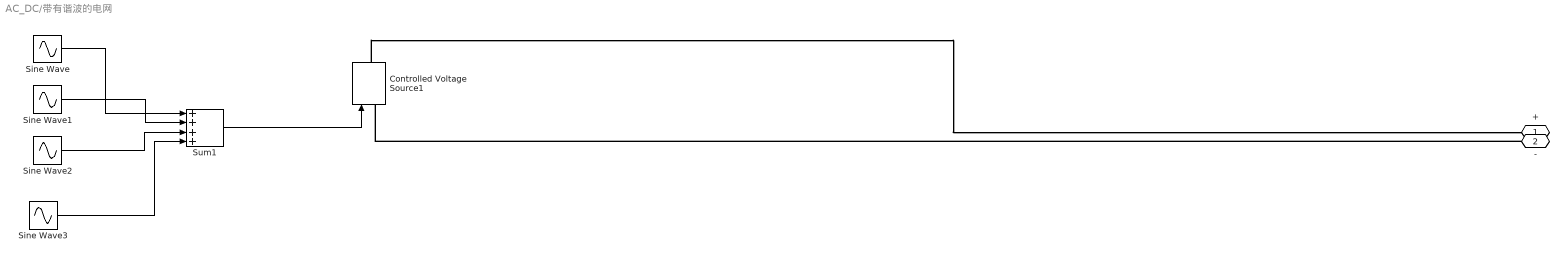
== system AC_DC/带有谐波的电网 ==
  Controlled Voltage Source1 : spsControlledVoltageSourceLib/Controlled Voltage Source  Initialize=off  Source_Type=AC  Amplitude=0  Phase=0  Frequency=0  Measurements=Voltage
  Sine Wave : Sin  Amplitude=32*sqrt(2)  Frequency=100*pi  SampleTime=0
  Sine Wave1 : Sin  Amplitude=0.04*32*sqrt(2)  Frequency=300*pi  SampleTime=0
  Sine Wave2 : Sin  Amplitude=0.03*32*sqrt(2)  Frequency=500*pi  SampleTime=0
  Sine Wave3 : Sin  Amplitude=0.02*32*sqrt(2)  Frequency=700*pi  SampleTime=0
  Sum1 : Sum  Inputs=++++
  + : PMIOPort  Side=Right
  - : PMIOPort  Port=2  Side=Left
  wires:
  Sum1/1 -> Controlled Voltage Source1/1
  Sine Wave1/1 -> Sum1/2
  Sine Wave/1 -> Sum1/1
  Sine Wave3/1 -> Sum1/4
  Sine Wave2/1 -> Sum1/3
  connections:
  -/RConn1 -- Controlled Voltage Source1/LConn1
  Controlled Voltage Source1/RConn1 -- +/RConn1

== matlab function AC_DC/MATLAB Function ==
  data: ua input; VT1 output; uanot input; ub input; ubnot input; t input; VT2 output; VT3 output; VT4 output
function [VT1, VT2, VT3, VT4] = fcn(ua, uanot, ub, ubnot, t)
% 输入：ua, uanot, ub, ubnot (PWM逻辑信号)
% 输入：t 时间
% 输出：VT1~VT4
% 逻辑：
% 0~0.4s：全部输出0
% 0.4~1.4s：正常输出
% 1.4s后：全部输出0

if (t >= 0 && t < 0.4) || t >=1.7
    % 0~0.4s 或 1.4s以后：全部输出 0.0（double类型）
    VT1 = 0.0;
    VT2 = 0.0;
    VT3 = 0.0;
    VT4 = 0.0;
else
    % 0.4s ~ 1.4s：正常输出PWM
    VT1 = double(ua);
    VT2 = double(uanot);
    VT3 = double(ub);
    VT4 = double(ubnot);
end

== matlab function AC_DC/MATLAB Function11 ==
  data: IGm_total input; IGm_clean output
function IGm_clean = Notch_100Hz_IGm(IGm_total)
    % 【动态窗口滑动平均滤波】专门消除100Hz纹波
    % 采样频率：20kHz，窗口长度：200点（20kHz/100Hz=200）
    % 核心改进：启动前200个点使用动态窗口，完全消除零值误差
    % 输入：IGm_total - 原始带纹波的电流信号
    % 输出：IGm_clean - 滤波后的平滑电流信号
    
    % 持久变量：仅在第一次调用时初始化，后续调用保留值
    persistent buffer   % 环形数据缓冲区
    persistent index    % 缓冲区当前写入索引
    persistent sum_buf  % 窗口内数据累加和（优化计算，避免循环求和）
    persistent sample_count % 已采样总点数（用于动态窗口判断）
    
    N = 200; % 固定窗口长度：100Hz纹波的精确零点
    
    % ====================== 初始化（仅第一次运行执行） ======================
    if isempty(buffer)
        buffer = zeros(1, N);  % 初始化环形缓冲区为全0
        index = 0;             % 索引从0开始
        sum_buf = 0;           % 累加和初始化为0
        sample_count = 0;      % 采样计数初始化为0
    end
    
    % ====================== 更新索引和计数 ======================
    sample_count = sample_count + 1; % 总采样数+1
    index = index + 1;
    if index > N
        index = 1; % 索引越界时回到起点，实现环形结构
    end
    
    % ====================== 核心滤波逻辑 ======================
    if sample_count <= N
        % ---------------------- 阶段1：动态窗口（前200个点） ----------------------
        % 不除以固定的200，而是除以当前已采样的点数
        % 第1个点：输出 = 第1个点 / 1
        % 第10个点：输出 = 前10个点和 / 10
        % ...
        % 第200个点：输出 = 前200个点和 / 200
        sum_buf = sum_buf + IGm_total;
        buffer(index) = IGm_total;
        IGm_clean = sum_buf / sample_count;
    else
        % ---------------------- 阶段2：标准滑动平均（200个点之后） ----------------------
        % 窗口已满，进入标准滑动模式
        % 减去最旧的采样值，加上最新的采样值
        sum_buf = sum_buf - buffer(index) + IGm_total;
        buffer(index) = IGm_total;
        IGm_clean = sum_buf / N;
    end
end

== matlab function AC_DC/MATLAB Function12 ==
  data: I_ref input; duty_out output; I_fb input
function duty_out = fcn(I_ref, I_fb)
%#codegen
% 同步Boost电流环PI控制器（带钳位抗饱和）
% 适配：20kHz采样、±5A电流传感器、占空比0.1~0.9安全范围
% 输入：
%   I_ref: 电压环输出的电流给定（对应你模型里电压环PI的输出）
%   I_fb: 电流反馈（对应你模型里经过-1增益后的IL信号）
% 输出：
%   duty_out: 最终占空比，直接接你模型里的1/z延迟模块

% 持久化变量：保存积分器状态，每个控制周期保留数值
persistent integral_val;
% 初始化：仅仿真启动的第一个控制周期执行1次
if isempty(integral_val)
    integral_val = 0;
end

% ==================== 1. 控制参数（和你原PI模块参数完全一致，可直接修改）====================
Kp = 0.5;       % 比例增益，和你原设置一致
Ki = 10;         % 积分增益，和你原设置一致
Ts = 5e-5;       % 20kHz控制周期，固定不变
% ==================== 2. 物理极限设置（核心抗饱和阈值）====================
DUTY_MAX = 3;  % 占空比上限，避免上下管直通
DUTY_MIN = -3;  % 占空比下限，杜绝轻载反向电流
I_SAT_LIMIT = 60.0; % 电流传感器饱和阈值，接近±5A量程提前触发保护

% ==================== 3. 误差计算 ====================
err = I_ref - I_fb;

% ==================== 4. 比例项输出 ====================
prop_out = Kp * err;

% ==================== 5. 核心抗饱和逻辑 ====================
% 5.1 积分项预计算
integral_inc = Ki * Ts * err;
integral_pre = integral_val + integral_inc;
% 5.2 预计算不饱和的PI输出
duty_pre = prop_out + integral_pre;

% 5.3 钳位抗饱和规则：
% 仅当输出在线性区、且电流未达到传感器饱和阈值时，才允许积分累加
% 同时加入反向积分放行规则，避免积分锁死
is_duty_linear = (duty_pre < DUTY_MAX) && (duty_pre > DUTY_MIN);
is_current_unsat = (abs(I_fb) < I_SAT_LIMIT);
is_integral_allow = is_duty_linear && is_current_unsat;
is_reverse_integral = (err > 0 && integral_pre < 0) || (err < 0 && integral_pre > 0);

if is_integral_allow || is_reverse_integral
    integral_val = integral_pre;
end

% ==================== 6. 最终占空比计算 + 硬限幅兜底 ====================
duty_out = prop_out + integral_val;
duty_out = min(max(duty_out, DUTY_MIN), DUTY_MAX);

== matlab function AC_DC/MATLAB Function13 ==
  data: ua input; VT1 output; uanot input; ub input; ubnot input; t input; VT2 output; VT3 output; VT4 output
function [VT1, VT2, VT3, VT4] = fcn(ua, uanot, ub, ubnot, t)
% 输入：ua, uanot, ub, ubnot (PWM逻辑信号)
% 输入：t 时间
% 输出：VT1~VT4
% 逻辑：
% 0~0.4s：全部输出0
% 0.4~1.4s：正常输出
% 1.4s后：全部输出0

if (t >= 0 && t < 0.4) || t >=1.7
    % 0~0.4s 或 1.4s以后：全部输出 0.0（double类型）
    VT1 = 0.0;
    VT2 = 0.0;
    VT3 = 0.0;
    VT4 = 0.0;
else
    % 0.4s ~ 1.4s：正常输出PWM
    VT1 = double(ua);
    VT2 = double(uanot);
    VT3 = double(ub);
    VT4 = double(ubnot);
end

== matlab function AC_DC/MATLAB Function14 ==
  data: i_error input; m output; t input
function m  = QPR_Current_Loop(i_error, t)
%#codegen
% 单相LCL整流器 电流环 多谐振QPR控制器【仅动态调整Kp】
% 动态Kp规则：
%   t < 0.4s：Kp=0.3（保持原值，开环前不工作）
%   0.4s ≤ t < 1.0s：Kp从10线性平滑降到0.3（延长下降时间）
%   t ≥ 1.0s：Kp=0.3（稳态小Kp，不放大纹波）
% 其他谐振项计算完全保留你原有的逻辑

%% ===================== 独立历史变量 =====================
persistent e1_1 e1_2 m1_1 m1_2  % 基波 n=1
persistent e3_1 e3_2 m3_1 m3_2  % 3次  n=3
persistent e5_1 e5_2 m5_1 m5_2  % 5次  n=5
persistent e7_1 e7_2 m7_1 m7_2  % 7次  n=7

%% ===================== 全局共用参数 =====================
Ts    = 1/20000;   % 采样周期

%% ===================== 各谐振项 独立参数（完全保留你的原值）=====================
% === 基波 50Hz (n=1) ===
Kr1 = 40;
wi1 = 6;
w01 = 100*pi;

% === 3次谐波 150Hz (n=3) ===
Kr3 = 100;
wi3 = 6;
w03 = 300*pi;

% === 5次谐波 250Hz (n=5) ===
Kr5 = 80;
wi5 = 6;
w05 = 500*pi;

% === 7次谐波 350Hz (n=7) ===
Kr7 = 60;
wi7 = 6;
w07 = 700*pi;

%% ===================== 初始化 =====================
if isempty(e1_1)
    e1_1=0;e1_2=0;m1_1=0;m1_2=0;
    e3_1=0;e3_2=0;m3_1=0;m3_2=0;
    e5_1=0;e5_2=0;m5_1=0;m5_2=0;
    e7_1=0;e7_2=0;m7_1=0;m7_2=0;
end

%% ===================== 核心：仅动态调整Kp（平滑曲线版本） =====================
t_start = 0.4;  % 开环时间
t_end   = 1;  % 结束时间
Kp_start = 0.3;  % 起始值
Kp_end   = 0.3; % 最终稳态值

if t < t_start
    Kp = 0.3;
elseif t >= t_start && t < t_end
    % 归一化时间 0~1
    tau = (t - t_start) / (t_end - t_start);
    % 余弦平滑曲线：开始慢、中间快、结束慢 → 无超调无冲击
    tau_smooth = 0.5 * (1 - cos(pi * tau));
    % 计算平滑Kp
    Kp = Kp_start - (Kp_start - Kp_end) * tau_smooth;
else
    Kp = Kp_end;
end
%% ===================== 1. 共用比例项（用动态Kp）=====================

m_p = Kp * i_error;

%% ===================== 2. 基波谐振项计算（完全保留你的逻辑）=====================
A1  = 2 * Kr1 * wi1;
B1  = 2 * wi1;
C1  = w01^2;
a0_1 = 4 + 2*B1*Ts + C1*Ts^2;
a1_1 = -8 + 2*C1*Ts^2;
a2_1 = 4 - 2*B1*Ts + C1*Ts^2;
b0_1 =  A1 * Ts;
b1_1 =  0;
b2_1 = -A1 * Ts;
m1 = (b0_1*i_error + b1_1*e1_1 + b2_1*e1_2 - a1_1*m1_1 - a2_1*m1_2) / a0_1;
% 更新
e1_2 = e1_1; e1_1 = i_error;
m1_2 = m1_1; m1_1 = m1;

%% ===================== 3. 3次谐波谐振项计算（完全保留你的逻辑）=====================
A3  = 2 * Kr3 * wi3;
B3  = 2 * wi3;
C3  = w03^2;
a0_3 = 4 + 2*B3*Ts + C3*Ts^2;
a1_3 = -8 + 2*C3*Ts^2;
a2_3 = 4 - 2*B3*Ts + C3*Ts^2;
b0_3 =  A3 * Ts;
b1_3 =  0;
b2_3 = -A3 * Ts;
m3 = (b0_3*i_error + b1_3*e3_1 + b2_3*e3_2 - a1_3*m3_1 - a2_3*m3_2) / a0_3;
% 更新
e3_2 = e3_1; e3_1 = i_error;
m3_2 = m3_1; m3_1 = m3;

%% ===================== 4. 5次谐波谐振项计算（完全保留你的逻辑）=====================
A5  = 2 * Kr5 * wi5;
B5  = 2 * wi5;
C5  = w05^2;
a0_5 = 4 + 2*B5*Ts + C5*Ts^2;
a1_5 = -8 + 2*C5*Ts^2;
a2_5 = 4 - 2*B5*Ts + C5*Ts^2;
b0_5 =  A5 * Ts;
b1_5 =  0;
b2_5 = -A5 * Ts;
m5 = (b0_5*i_error + b1_5*e5_1 + b2_5*e5_2 - a1_5*m5_1 - a2_5*m5_2) / a0_5;
% 更新
e5_2 = e5_1; e5_1 = i_error;
m5_2 = m5_1; m5_1 = m5;

%% ===================== 5. 7次谐波谐振项计算（完全保留你的逻辑）=====================
A7  = 2 * Kr7 * wi7;
B7  = 2 * wi7;
C7  = w07^2;
a0_7 = 4 + 2*B7*Ts + C7*Ts^2;
a1_7 = -8 + 2*C7*Ts^2;
a2_7 = 4 - 2*B7*Ts + C7*Ts^2;
b0_7 =  A7 * Ts;
b1_7 =  0;
b2_7 = -A7 * Ts;
m7 = (b0_7*i_error + b1_7*e7_1 + b2_7*e7_2 - a1_7*m7_1 - a2_7*m7_2) / a0_7;
% 更新
e7_2 = e7_1; e7_1 = i_error;
m7_2 = m7_1; m7_1 = m7;

%% ===================== 总输出叠加 =====================
m = m_p + m1 + m3 + m5 + m7;

end

== matlab function AC_DC/MATLAB Function17 ==
  data: IGm_total input; IGm_clean output
function IGm_clean = Notch_100Hz_IGm(IGm_total)
    % 【动态窗口滑动平均滤波】专门消除100Hz纹波
    % 采样频率：20kHz，窗口长度：200点（20kHz/100Hz=200）
    % 核心改进：启动前200个点使用动态窗口，完全消除零值误差
    % 输入：IGm_total - 原始带纹波的电流信号
    % 输出：IGm_clean - 滤波后的平滑电流信号
    
    % 持久变量：仅在第一次调用时初始化，后续调用保留值
    persistent buffer   % 环形数据缓冲区
    persistent index    % 缓冲区当前写入索引
    persistent sum_buf  % 窗口内数据累加和（优化计算，避免循环求和）
    persistent sample_count % 已采样总点数（用于动态窗口判断）
    
    N = 200; % 固定窗口长度：100Hz纹波的精确零点
    
    % ====================== 初始化（仅第一次运行执行） ======================
    if isempty(buffer)
        buffer = zeros(1, N);  % 初始化环形缓冲区为全0
        index = 0;             % 索引从0开始
        sum_buf = 0;           % 累加和初始化为0
        sample_count = 0;      % 采样计数初始化为0
    end
    
    % ====================== 更新索引和计数 ======================
    sample_count = sample_count + 1; % 总采样数+1
    index = index + 1;
    if index > N
        index = 1; % 索引越界时回到起点，实现环形结构
    end
    
    % ====================== 核心滤波逻辑 ======================
    if sample_count <= N
        % ---------------------- 阶段1：动态窗口（前200个点） ----------------------
        % 不除以固定的200，而是除以当前已采样的点数
        % 第1个点：输出 = 第1个点 / 1
        % 第10个点：输出 = 前10个点和 / 10
        % ...
        % 第200个点：输出 = 前200个点和 / 200
        sum_buf = sum_buf + IGm_total;
        buffer(index) = IGm_total;
        IGm_clean = sum_buf / sample_count;
    else
        % ---------------------- 阶段2：标准滑动平均（200个点之后） ----------------------
        % 窗口已满，进入标准滑动模式
        % 减去最旧的采样值，加上最新的采样值
        sum_buf = sum_buf - buffer(index) + IGm_total;
        buffer(index) = IGm_total;
        IGm_clean = sum_buf / N;
    end
end

== matlab function AC_DC/MATLAB Function18 ==
  data: I_ref input; duty_out output; I_fb input
function duty_out = fcn(I_ref, I_fb)
%#codegen
% 同步Boost电流环PI控制器（带钳位抗饱和）
% 适配：20kHz采样、±5A电流传感器、占空比0.1~0.9安全范围
% 输入：
%   I_ref: 电压环输出的电流给定（对应你模型里电压环PI的输出）
%   I_fb: 电流反馈（对应你模型里经过-1增益后的IL信号）
% 输出：
%   duty_out: 最终占空比，直接接你模型里的1/z延迟模块

% 持久化变量：保存积分器状态，每个控制周期保留数值
persistent integral_val;
% 初始化：仅仿真启动的第一个控制周期执行1次
if isempty(integral_val)
    integral_val = 0;
end

% ==================== 1. 控制参数（和你原PI模块参数完全一致，可直接修改）====================
Kp = 0.5;       % 比例增益，和你原设置一致
Ki = 10;         % 积分增益，和你原设置一致
Ts = 5e-5;       % 20kHz控制周期，固定不变
% ==================== 2. 物理极限设置（核心抗饱和阈值）====================
DUTY_MAX = 4;  % 占空比上限，避免上下管直通
DUTY_MIN = -4;  % 占空比下限，杜绝轻载反向电流
I_SAT_LIMIT = 60.0; % 电流传感器饱和阈值，接近±5A量程提前触发保护

% ==================== 3. 误差计算 ====================
err = I_ref - I_fb;

% ==================== 4. 比例项输出 ====================
prop_out = Kp * err;

% ==================== 5. 核心抗饱和逻辑 ====================
% 5.1 积分项预计算
integral_inc = Ki * Ts * err;
integral_pre = integral_val + integral_inc;
% 5.2 预计算不饱和的PI输出
duty_pre = prop_out + integral_pre;

% 5.3 钳位抗饱和规则：
% 仅当输出在线性区、且电流未达到传感器饱和阈值时，才允许积分累加
% 同时加入反向积分放行规则，避免积分锁死
is_duty_linear = (duty_pre < DUTY_MAX) && (duty_pre > DUTY_MIN);
is_current_unsat = (abs(I_fb) < I_SAT_LIMIT);
is_integral_allow = is_duty_linear && is_current_unsat;
is_reverse_integral = (err > 0 && integral_pre < 0) || (err < 0 && integral_pre > 0);

if is_integral_allow || is_reverse_integral
    integral_val = integral_pre;
end

% ==================== 6. 最终占空比计算 + 硬限幅兜底 ====================
duty_out = prop_out + integral_val;
duty_out = min(max(duty_out, DUTY_MIN), DUTY_MAX);

== matlab function AC_DC/MATLAB Function21 ==
  data: in1 input; out1 output; in2 input; in3 input; in4 input; in5 input; in6 input; in7 input; t input; out2 output; out3 output; out4 output; out5 output; out6 output; out7 output
function [out1, out2, out3, out4, out5, out6, out7] = fcn(in1, in2, in3, in4, in5, in6, in7, t)
% 输入：
% in1~in7 : 7路采样信号
% t       : 仿真时间 (需连接Clock模块)
% 输出：
% out1~out7: 0.4秒前全为0，0.4秒后输出采样值

% ====================== 核心判断（只有一行） ======================
if t >= 0.4
    % 时间到：输出采样值
    out1 = in1;
    out2 = in2;
    out3 = in3;
    out4 = in4;
    out5 = in5;
    out6 = in6;
    out7 = in7;
else
    % 时间未到：全部输出0
    out1 = 0;
    out2 = 0;
    out3 = 0;
    out4 = 0;
    out5 = 0;
    out6 = 0;
    out7 = 0;
end
